simulink model "nolinear_system"  (R2022a)
settings: Solver=ode15s  StartTime=0.0  StopTime=10.0
values from neighbouring files (symbols this model uses):
  a1 = -z2/z1    (= 0.769230769231)    [params.m]    (also in params_nolinear_system.m = -z2/z1)
  a2 = z2*eps/z1    (= 2.331002331)    [params.m]    (also in params_nolinear_system.m = z2*eps/z1)
  a3 = z3/z1    (= 2.47815294211)    [params.m]    (also in params_nolinear_system.m = z3/z1)
  a4 = k/z1    (= 1.09686889935)    [params.m]    (also in params_nolinear_system.m = k/z1)
  b1 = -z4/z5    (= 0.822324878959)    [params.m]    (also in params_nolinear_system.m = -z4/z5)
  b2 = z7/(eps*z5)    (= 8.06700706259)    [params.m]    (also in params_nolinear_system.m = z7/(eps*z5))
  b3 = z6/z5    (= 0.963345768584)    [params.m]    (also in params_nolinear_system.m = z6/z5)
  b4 = -k/z5    (= 0.426391767402)    [params.m]    (also in params_nolinear_system.m = -k/z5)
  K = [1 1 1 1]    [params.m]
undefined symbols (not defined in the file or in its folder): magnitude
settings Model: Creator=epyur  LastModifiedBy=epyur
settings SolverCC: ZeroCrossControl=DisableAll
settings DebuggingCC: AlgebraicLoopMsg=none

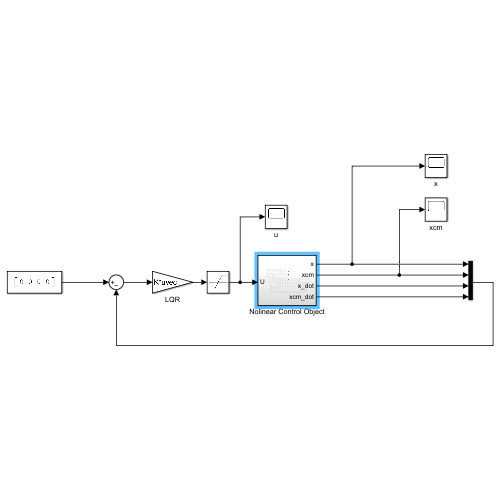
[thumbnail: Simulink's stored preview of the top-level diagram]
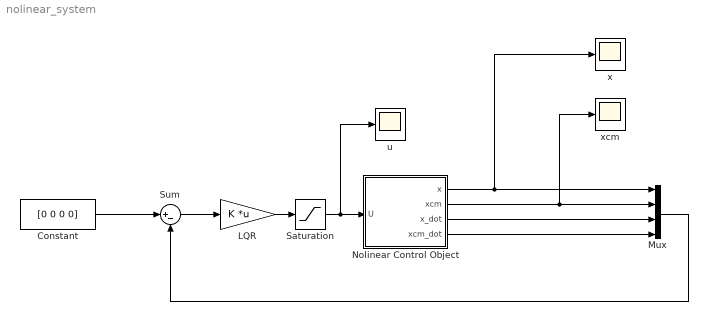
== system nolinear_system ==
  Constant : Constant  Value=[0 0 0 0]  VectorParams1D=off
  LQR : Gain  Gain=K  Multiplication=Matrix(K*u) (u vector)
  Mux : Mux
  Nolinear Control Object : Subsystem
  Saturation : Saturate  UpperLimit=24  LowerLimit=-24
  Sum : Sum  Inputs=|+-
  u : Scope
  x : Scope
  xcm : Scope
  wires:
  Nolinear Control Object/1(x) -> x/1, Mux/1
  Nolinear Control Object/3(x_dot) -> Mux/3
  Nolinear Control Object/4(xcm_dot) -> Mux/4
  Mux/1 -> Sum/2
  Constant/1 -> Sum/1
  Sum/1 -> LQR/1
  LQR/1 -> Saturation/1
  Saturation/1 -> u/1, Nolinear Control Object/1(U)
  Nolinear Control Object/2(xcm) -> xcm/1, Mux/2

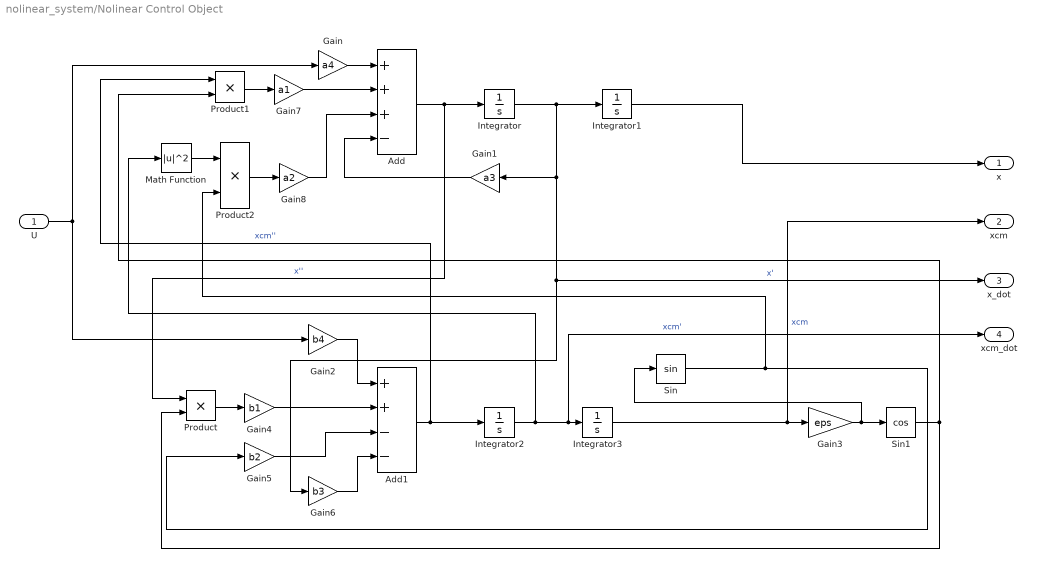
== system nolinear_system/Nolinear Control Object ==
  U : Inport
  Add : Sum  Inputs=+++-
  Add1 : Sum  Inputs=++--
  Gain : Gain  Gain=a4
  Gain1 : Gain  Gain=a3
  Gain2 : Gain  Gain=b4
  Gain3 : Gain  Gain=eps
  Gain4 : Gain  Gain=b1
  Gain5 : Gain  Gain=b2
  Gain6 : Gain  Gain=b3
  Gain7 : Gain  Gain=a1
  Gain8 : Gain  Gain=a2
  Integrator : Integrator
  Integrator1 : Integrator
  Integrator2 : Integrator
  Integrator3 : Integrator  InitialCondition=-0.144
  Math Function : Math  Operator=magnitude^2
  Product : Product
  Product1 : Product
  Product2 : Product
  Sin : Trigonometry
  Sin1 : Trigonometry  Operator=cos
  x : Outport
  xcm : Outport  Port=2
  x_dot : Outport  Port=3
  xcm_dot : Outport  Port=4
  wires:
  Add/1 -> Integrator/1, Product/1  "x''"
  Integrator/1 -> Gain6/1, x_dot/1, Gain1/1, Integrator1/1  "x'"
  Gain/1 -> Add/1
  U/1 -> Gain/1, Gain2/1
  Gain1/1 -> Add/4
  Gain2/1 -> Add1/1
  Add1/1 -> Integrator2/1, Product1/1  "xcm''"
  Integrator2/1 -> Math Function/1, xcm_dot/1, Integrator3/1  "xcm'"
  Integrator3/1 -> xcm/1, Gain3/1  "xcm"
  Gain3/1 -> Sin/1, Sin1/1
  Gain4/1 -> Add1/2
  Product/1 -> Gain4/1
  Sin1/1 -> Product1/2, Product/2
  Gain5/1 -> Add1/3
  Sin/1 -> Product2/2, Gain5/1
  Gain6/1 -> Add1/4
  Gain7/1 -> Add/2
  Product1/1 -> Gain7/1
  Math Function/1 -> Product2/1
  Product2/1 -> Gain8/1
  Gain8/1 -> Add/3
  Integrator1/1 -> x/1
